simulink model "FullVehicleModel_ABS_ESP"  (R2019a)
settings: Solver=ode23s  StartTime=0.0  StopTime=t_f  MaxStep=0.1  RelTol=1e-3
values from neighbouring files (symbols this model uses):
  acc_US_test = 0    [mainVehicleModel.m]
  auxiliary_data = block.DialogPrm(3).Data    [FullVehicleModel_V3_sfun.m]    (also in mainVehicleModel.m = getAuxiliaryDataStruct())
  curv_akermann = 0    [mainVehicleModel.m]
  hv = 0.5    [mainVehicleModel.m]
  init_conditions_data = getInitialConditionsDataStruct( V_init )    [mainVehicleModel.m]
  lambda1_th = 0.2    [mainVehicleModel.m]
  lambda2_th = 0.1    [mainVehicleModel.m]
  maneuver_flag = 4    [mainVehicleModel.m]
  parametri_ABS = para    [ABSParameters.m]    (also in mainVehicleModel.m = ABSParameters(getVehicleDataStruct()))
  rho_off = 0.9    [mainVehicleModel.m]
  rho_on = 1.02    [mainVehicleModel.m]
  t_brake = t_f+1    (= 61)    [mainVehicleModel.m]
  Tb_dot_max = 5000    [mainVehicleModel.m]
  V_init = 50    [mainVehicleModel.m]
  v_on = 2.5    [mainVehicleModel.m]
  v_stop = 0.1    [mainVehicleModel.m]
  vehicle_data = block.DialogPrm(1).Data    [FullVehicleModel_V3_sfun.m]    (also in mainVehicleModel.m = getVehicleDataStruct())
undefined symbols (not defined in the file or in its folder): magnitude, sigbuilder_block
libraries: simulink x6, dspsigops x4
(part 2 of 2)

== stateflow chart FullVehicleModel_ABS_ESP/ABS and Wheel torque generation/ABS Rear Right Wheel/Subsystem/Activation and Deactivation Logic1 ==
  state High_Speed_ON
    entry: Tb_select = 2;
    entry: ABS_ON = true;
  state High_Speed_OFF
    entry: Tb_select = 1;
    entry: ABS_ON = false;
  state Low_Speed_ON
    entry: Tb_select = 3;
    entry: ABS_ON = true;
  state Low_Speed_OFF
    entry: Tb_select = 1;
    entry: ABS_ON = false;
  High_Speed_OFF -> High_Speed_ON [order 1] : [lambda > lambda1_th - ((lambda1_th - lambda2_th)/1500)*Tb_dot && ...
      |  Tb_Dr > rho_on*Tb_Ctrl && ...
      |  v > v_on]
  (default) -> High_Speed_OFF : {Tb_select = 1;}
  High_Speed_ON -> High_Speed_OFF [order 1] : [Tb_Dr < rho_off*Tb_Ctrl]
  High_Speed_OFF -> Low_Speed_OFF [order 2] : [v < v_on -hv]
  Low_Speed_OFF -> High_Speed_OFF : [v > v_on +hv]
  High_Speed_ON -> Low_Speed_ON [order 2] : [v < v_on]
  Low_Speed_ON -> Low_Speed_OFF : [v < v_stop || Tb_Dr < rho_off*Tb_LPF]
  data: Tb_select output; Tb_Dr input; Tb_Ctrl input; v input; Tb_dot input; Tb_dot_max parameter; v_on parameter; rho_on parameter; Tb_LPF input; lambda input; lambda1_th parameter; v_stop parameter; hv parameter; rho_off parameter; ABS_ON output; lambda2_th parameter

== matlab function FullVehicleModel_ABS_ESP/ABS and Wheel torque generation/ABS Front Left Wheel/MATLAB Function ==
  data: lambda input; RHS output; Tb input; v input; vehicle_data parameter; Fz input
function RHS = lambdaDyn(lambda,Tb,v,vehicle_data,Fz)

omega = (1-lambda)*v/vehicle_data.front_wheel.Rf;

Psi = (vehicle_data.front_wheel.Rf+vehicle_data.front_wheel.iwd_f/(vehicle_data.front_wheel.iwd_f*vehicle_data.vehicle.m)*(1-lambda))*Fz*1.5*burckhardt(lambda,1);

if omega<=1
    RHS=0;
else
    RHS=-((1-lambda)/(vehicle_data.front_wheel.iwd_f*omega))*(Psi-Tb);
end

end

== stateflow chart FullVehicleModel_ABS_ESP/ABS and Wheel torque generation/ABS Front Left Wheel/Subsystem/Activation and Deactivation Logic1 ==
  state High_Speed_ON
    entry: Tb_select = 2;
    entry: ABS_ON = true;
  state High_Speed_OFF
    entry: Tb_select = 1;
    entry: ABS_ON = false;
  state Low_Speed_ON
    entry: Tb_select = 3;
    entry: ABS_ON = true;
  state Low_Speed_OFF
    entry: Tb_select = 1;
    entry: ABS_ON = false;
  High_Speed_OFF -> High_Speed_ON [order 1] : [lambda > lambda1_th - ((lambda1_th - lambda2_th)/3000)*Tb_dot && ...
      |  Tb_Dr > rho_on*Tb_Ctrl && ...
      |  v > v_on]
  (default) -> High_Speed_OFF : {Tb_select = 1;}
  High_Speed_ON -> High_Speed_OFF [order 1] : [Tb_Dr < rho_off*Tb_Ctrl]
  High_Speed_OFF -> Low_Speed_OFF [order 2] : [v < v_on -hv]
  Low_Speed_OFF -> High_Speed_OFF : [v > v_on +hv]
  High_Speed_ON -> Low_Speed_ON [order 2] : [v < v_on]
  Low_Speed_ON -> Low_Speed_OFF : [v < v_stop || Tb_Dr < rho_off*Tb_LPF]
  data: Tb_select output; Tb_Dr input; Tb_Ctrl input; v input; Tb_dot input; Tb_dot_max parameter; v_on parameter; rho_on parameter; Tb_LPF input; lambda input; lambda1_th parameter; v_stop parameter; hv parameter; rho_off parameter; ABS_ON output; lambda2_th parameter

== matlab function FullVehicleModel_ABS_ESP/ABS and Wheel torque generation/ABS Rear Left Wheel/Subsystem/MATLAB Function ==
  data: Tb input; Tb_Ctrl output; t_brake parameter
function Tb_Ctrl = biasedTb(Tb,t_brake)


Tb_Ctrl = (3-t_brake)*160+Tb;
end

== matlab function FullVehicleModel_ABS_ESP/ABS and Wheel torque generation/ABS Rear Right Wheel/MATLAB Function1 ==
  data: lambda input; ex output; Tb_dot input; parametri_ABS parameter
function ex = lambdacheck(lambda,Tb_dot,parametri_ABS)

if lambda > parametri_ABS.lambda1_th - ((parametri_ABS.lambda1_th - parametri_ABS.lambda2_th)/7000)*Tb_dot
    ex=1;
else
    ex=0;
end

== matlab function FullVehicleModel_ABS_ESP/ABS and Wheel torque generation/ABS Rear Right Wheel/Subsystem/MATLAB Function ==
  data: Tb input; Tb_Ctrl output; t_brake parameter
function Tb_Ctrl = biasedTb(Tb,t_brake)


Tb_Ctrl = (3-t_brake)*160+Tb;
end
